simulink subsystem "kalman_position"  (R2025b)
settings: Solver=VariableStepAuto  StartTime=0.0  StopTime=10.0  RelTol=1e-3
undefined symbols (not defined in the file or in its folder): DiscIntNeverNeededParam
settings Model: Creator=schwmaxi  LastModifiedBy=schwmaxi

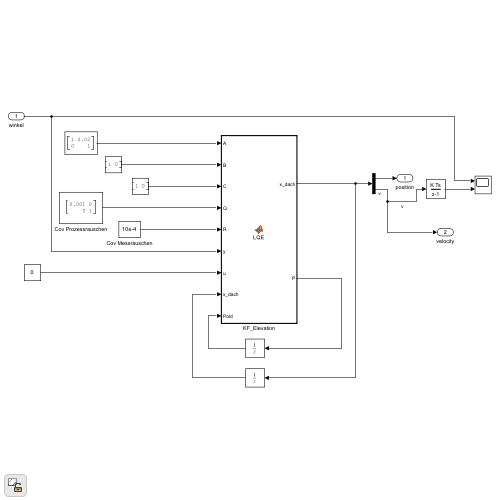
[thumbnail: Simulink's stored preview of the top-level diagram]
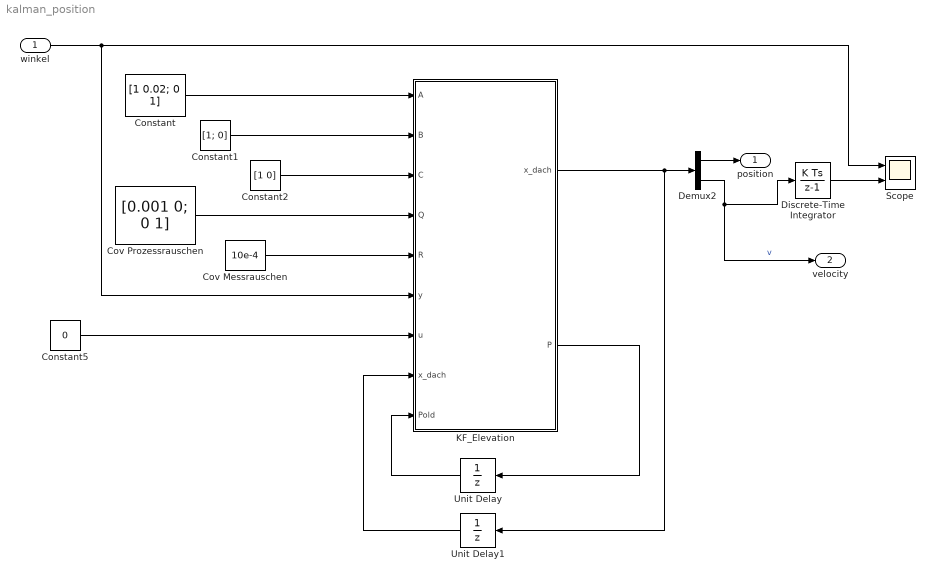
== system kalman_position ==
  winkel : Inport
  Constant : Constant  Value=[1 0.02; 0 1]
  Constant1 : Constant  Value=[1; 0]
  Constant2 : Constant  Value=[1 0]  VectorParams1D=off
  Constant5 : Constant  Value=0
  Cov Messrauschen : Constant  Value=10e-4
  Cov Prozessrauschen : Constant  Value=[0.001 0; 0 1]
  Demux2 : Demux  Outputs=2
  Discrete-Time Integrator : DiscreteIntegrator  SampleTime=-1  ICPrevOutput=DiscIntNeverNeededParam  ICPrevScaledInput=DiscIntNeverNeededParam
  KF_Elevation : MATLAB Function  TreatAsAtomicUnit=on
  Scope : Scope  NumInputPorts=2
      settings: ActiveDisplayYMinimum=-0.02594686015874631  ActiveDisplayYMaximum=0.25963655751257553  DataLoggingVariableName=ScopeData8
  Unit Delay : UnitDelay  InitialCondition=1 * eye(2, 2)  SampleTime=-1  HasFrameUpgradeWarning=on
  Unit Delay1 : UnitDelay  InitialCondition=[0; 0]  SampleTime=-1  HasFrameUpgradeWarning=on
  position : Outport
  velocity : Outport  Port=2
  wires:
  Unit Delay1/1 -> KF_Elevation/8("x_dach ")
  Constant2/1 -> KF_Elevation/3(C)
  KF_Elevation/2(P) -> Unit Delay/1
  Constant1/1 -> KF_Elevation/2(B)
  KF_Elevation/1(x_dach) -> Demux2/1, Unit Delay1/1
  Unit Delay/1 -> KF_Elevation/9(Pold)
  winkel/1 -> Scope/1, KF_Elevation/6(y)
  Cov Messrauschen/1 -> KF_Elevation/5(R)
  Demux2/1 -> position/1
  Constant5/1 -> KF_Elevation/7(u)
  Constant/1 -> KF_Elevation/1(A)
  Cov Prozessrauschen/1 -> KF_Elevation/4(Q)
  Discrete-Time Integrator/1 -> Scope/2
  Demux2/2 -> velocity/1, Discrete-Time Integrator/1  "v"

== matlab function kalman_position/KF_Elevation ==
  settings: updateMethod=DISCRETE
  data: A input; B input; x_dach output; C input; Q input; R input; y input; u input; x_dach input; P output; Pold input
% LQE
% DDMLTS
% Universität Augsburg
% Lehrstuhl Regelungstechnik
% F. Friedrich, 02.02.2022
function [x_dach,P]  = LQE(A,B,C,Q,R,y,u,x_dach,Pold)

% PRÄDIKTION:
% 1. Schritt: Kovarianzmatrix prädizieren:
P_pred = A * Pold * A' + Q;

% 2. Schritt: Parameterschätzung prädizieren:
x_pred = A * x_dach + B *u;

% KORREKTUR:
% 3. Schritt: Verstärkung korrigieren
K = P_pred * C' / (R + C * P_pred * C');

% 4. Schritt: Parameterschätzung korrigieren
x_dach = x_pred + K * (y - C * x_pred);

% 5. Schritt: Kovarianzmatrix korrigieren
P = (eye(size(P_pred)) - K * C) * P_pred * (eye(size(P_pred)) - K * C)' + K * R * K';

end
